simulink subsystem "Lib_AlignAsyncSignal"  (R2023b)
settings: Solver=VariableStepAuto  StartTime=0.0  StopTime=10.0  RelTol=1e-3
libraries: hdlsllib x1
settings Model: Creator=naxin  LastModifiedBy=naxin

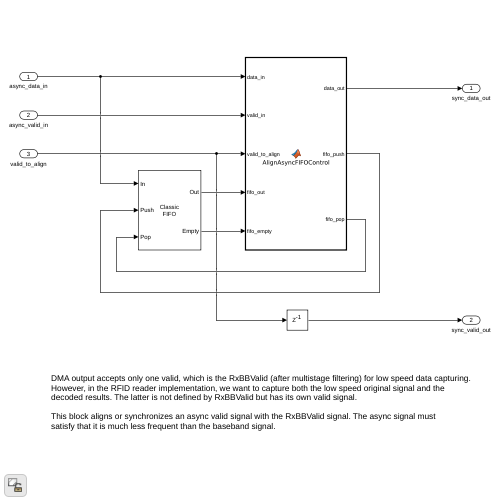
[thumbnail: Simulink's stored preview of the top-level diagram]
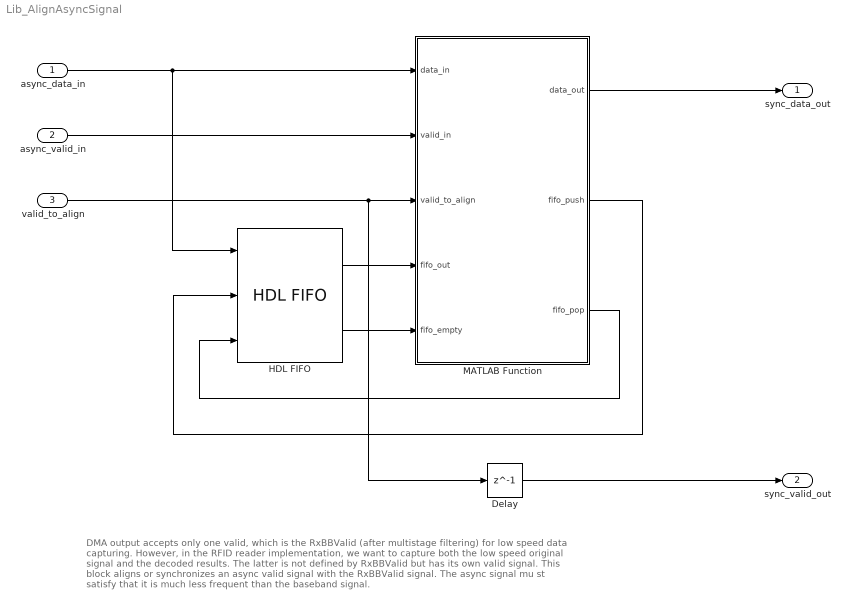
== system Lib_AlignAsyncSignal ==
  note: DMA output accepts only one valid, which is the RxBBValid (after multistage filtering) for low speed data capturing. However, in the RFID reader implementation, we want to capture both the low speed original signal and the decoded results. The latter is not defined by RxBBValid but has its own valid signal.
      |
      | This block aligns or synchronizes an async valid signal with the RxBBValid signal. The async signal mu st
      | satisfy that it is much less frequent than the baseband signal.
  async_data_in : Inport
  async_valid_in : Inport  Port=2
  valid_to_align : Inport  Port=3
  Delay : Delay  DelayLength=1  InitialCondition=false
  HDL FIFO : hdlsllib/HDL RAMs/HDL FIFO  fifo_size=256  mode=Classic  ratio=1  push_msg=Warning  pop_msg=Warning  show_empty=on  show_full=off  show_num=off  LabelModeActiveChoice_Mode=Classic  rst_port=off
  MATLAB Function : MATLAB Function  TreatAsAtomicUnit=on
  sync_data_out : Outport
  sync_valid_out : Outport  Port=2
  wires:
  async_valid_in/1 -> MATLAB Function/2(valid_in)
  HDL FIFO/2 -> MATLAB Function/5(fifo_empty)
  MATLAB Function/3(fifo_pop) -> HDL FIFO/3
  HDL FIFO/1 -> MATLAB Function/4(fifo_out)
  async_data_in/1 -> HDL FIFO/1, MATLAB Function/1(data_in)
  valid_to_align/1 -> MATLAB Function/3(valid_to_align), Delay/1
  MATLAB Function/2(fifo_push) -> HDL FIFO/2
  Delay/1 -> sync_valid_out/1
  MATLAB Function/1(data_out) -> sync_data_out/1

== matlab function Lib_AlignAsyncSignal/MATLAB Function ==
  settings: fimath=fimath('RoundingMethod', 'Floor','OverflowAction', 'Wrap','ProductMode', 'FullPrecision', 'SumMode', 'FullPrecision')
  data: data_in input; data_out output; valid_in input; valid_to_align input; fifo_out input; fifo_empty input; fifo_push output; fifo_pop output
function [data_out, fifo_push, fifo_pop] = AlignAsyncFIFOControl(data_in, valid_in, valid_to_align, fifo_out, fifo_empty)
% This is the main control function. We use a FIFO to store the async data.
%  Since the output of the FIFO happens one step after a pop true, we must
%  assert all data_out work the same way with this.
% output:
%    `data_out`: data output signal, happens one sample delay after `valid_to_align`
%    `fifo_push`: control signal of fifo, push
%    `fifo_pop`: control signal of fifo, pop
% input:
%    `data_in`: data input, the data needed to be aligned
%    `valid_in`: valid input signal, together with data_in
%    `valid_to_align`: valid signal the above two need to align
%    `fifo_out`: fifo output data
%    `fifo_empty`: fifo monitor signal, empty
%
% Our actions and what to output are determined by the three input logic,
%  i.e., valid_in, valid_to_align, fifo_empty. The specific actions are
%  shown in the following table:
% | valid_in  | valid_to_align |  nonempty |   Actions
% |     0     |        0       |     0     | no push, no pop, output none
% |     0     |        0       |     1     | no push, no pop, output none
% |     0     |        1       |     0     | no push, no pop, output none
% |     0     |        1       |     1     | no push, pop and output fifo
% |     1     |        0       |     0     | push, no pop and output none
% |     1     |        0       |     1     | push, no pop and output none
% |     1     |        1       |     0     | no push, no pop, output temp store
% |     1     |        1       |     1     | push, pop and output fifo
% 
% Register logic can be simply represented by the first step below.
% In order to implement this, we first check `valid_to_align`. If it is
%  false, then we definitely don't pop and output none. Then we perform
%  actions by checking `valid_in` and `fifo_empty`.
%
%#codegen
    persistent output_none_reg output_fifo_reg instant_store_reg;
    if isempty(output_none_reg)
        output_none_reg   = true;
        output_fifo_reg   = true;
        instant_store_reg = zeros('like', data_in);
    end
    
    %% 0. take registers
    output_none = output_none_reg;
    output_fifo = output_fifo_reg;
    store_data  = instant_store_reg;

    %% 1. determine what to output now
    if output_none
        data_out = zeros('like', data_in);
    elseif output_fifo
        data_out = fifo_out;
    else
        data_out = store_data;
    end

    %% 2. determine what to do
    if ~valid_to_align
        fifo_push = valid_in;
        fifo_pop  = false;
        output_none_reg   = true;
        output_fifo_reg   = true;
        instant_store_reg = zeros('like', data_in);
    else
        fifo_push = valid_in & ~fifo_empty;
        fifo_pop  = ~fifo_empty;
        if ~fifo_empty
            output_none_reg   = false;
            output_fifo_reg   = true;
            instant_store_reg = zeros('like', data_in);
        elseif valid_in
            output_none_reg   = false;
            output_fifo_reg   = false;
            instant_store_reg = data_in;
        else
            output_none_reg   = true;
            output_fifo_reg   = true;
            instant_store_reg = zeros('like', data_in);
        end
    end
end
